simulink model "Sistema_Seguimiento_Final"  (R2016a)
settings: Solver=VariableStepAuto  StartTime=0.0  StopTime=30  RelTol=1e-3
values from neighbouring files (symbols this model uses):
  K = acker(Ahat, Bhat ,PLC)    [AuxAcker.m]    (also in MiFinal_6_12_2024.m)
undefined symbols (not defined in the file or in its folder): A, C
settings Model: Creator=Abel  LastModifiedBy=Abel

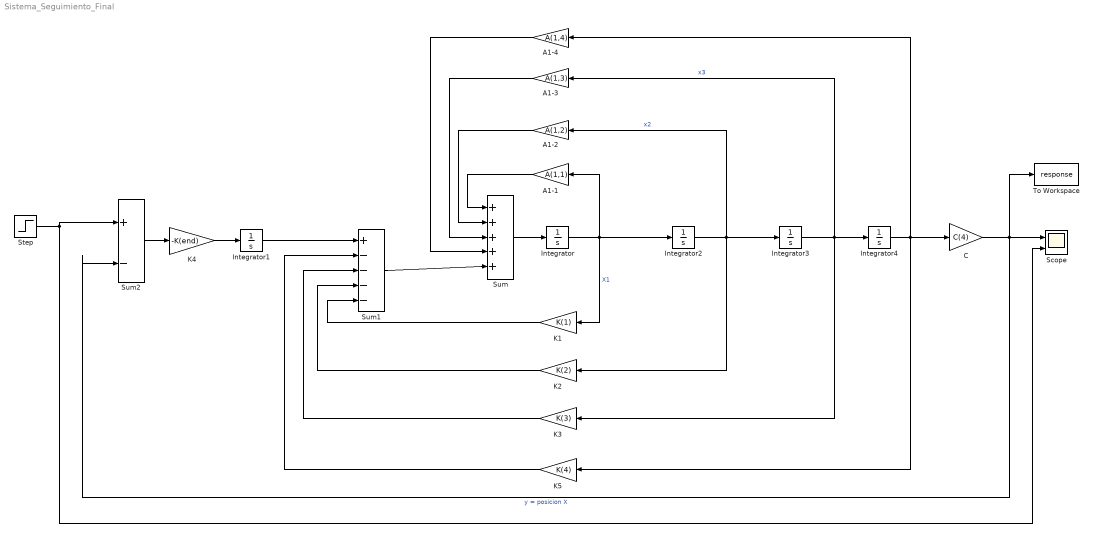
== system Sistema_Seguimiento_Final ==
  A1-1 : Gain  Gain=A(1,1)
  A1-2 : Gain  Gain=A(1,2)
  A1-3 : Gain  Gain=A(1,3)
  A1-4 : Gain  Gain=A(1,4)
  C : Gain  Gain=C(4)
  Integrator{,1..4} (5 alike) : Integrator
  K1 : Gain  Gain=K(1)
  K2 : Gain  Gain=K(2)
  K3 : Gain  Gain=K(3)
  K4 : Gain  Gain=-K(end)
  K5 : Gain  Gain=K(4)
  Scope : Scope  NumInputPorts=2
  Step : Step  Time=0  SampleTime=0
  Sum : Sum  Inputs=|+|+|+|+||+|
  Sum1 : Sum  Inputs=|+|-|-|-|-|
  Sum2 : Sum  Inputs=|+|-|
  To Workspace : ToWorkspace  VariableName=response  SaveFormat=Timeseries  SampleTime=-1
      settings: Save2DSignal=2-D array (concatenate along first dimension)
  wires:
  Integrator/1 -> K1/1, Integrator2/1, A1-1/1  "X1"
  Sum/1 -> Integrator/1
  A1-1/1 -> Sum/1
  A1-2/1 -> Sum/2
  Integrator2/1 -> K2/1, Integrator3/1, A1-2/1  "x2"
  Sum2/1 -> K4/1
  Integrator3/1 -> K3/1, Integrator4/1, A1-3/1  "x3"
  A1-3/1 -> Sum/3
  K4/1 -> Integrator1/1
  Integrator1/1 -> Sum1/1
  Sum1/1 -> Sum/5
  Step/1 -> Sum2/1, Scope/2
  A1-4/1 -> Sum/4
  Integrator4/1 -> A1-4/1, C/1, K5/1
  K1/1 -> Sum1/5
  K2/1 -> Sum1/4
  K3/1 -> Sum1/3
  K5/1 -> Sum1/2
  C/1 -> Sum2/2, To Workspace/1, Scope/1  "y = posicion X"
